simulink model "embedded_zeros"  (Simulink 7.6)
settings: Solver=FixedStepDiscrete  StartTime=0.0  StopTime=10.0  FixedStep=1  RelTol=1e-3
settings Model: Creator=Administrator  LastModifiedBy=c2wt
settings OptimizationCC: InitFltsAndDblsToZero=on
settings DebuggingCC: SaveWithParameterizedLinksMsg=none  StrictBusMsg=Warning
settings SFSimCC: SimParseCustomCode=off

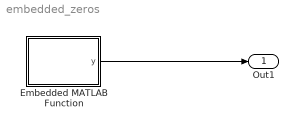
== system embedded_zeros ==
  Embedded MATLAB Function : Stateflow chart  TreatAsAtomicUnit=on
  Out1 : Outport  OutDataTypeStr=int32  PortDimensions=[3 3]
  wires:
  Embedded MATLAB Function/1(y) -> Out1/1

== matlab function Embedded MATLAB Function ==
  data: y output int32 size=[3 3]
function y = fcn()
% This block supports the Embedded MATLAB subset.
% See the help menu for details. 

y = zeros(3,3,'int32')

y = y + 1
